simulink model "testNoise"  (R2023b)
settings: Solver=VariableStepAuto  StartTime=0.0  StopTime=10.0  RelTol=1e-3
libraries: simulink x1
settings Model: Creator=grouleau  LastModifiedBy=grouleau

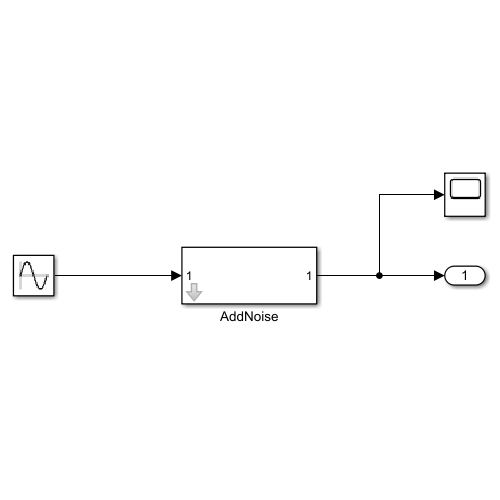
[thumbnail: Simulink's stored preview of the top-level diagram]
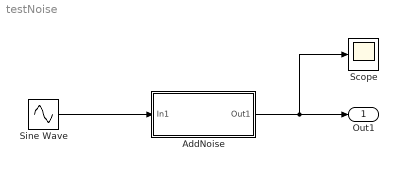
== system testNoise ==
  AddNoise : Subsystem  mask{choice=Random}
      mask prompts: choice "Type of noise"
      mask TypeOptions choice: Random | Pulse | Sequence
  Scope : Scope
  Sine Wave : Sin  Amplitude=5  SampleTime=0
  Out1 : Outport
  wires:
  AddNoise/1(Out1) -> Scope/1, Out1/1
  Sine Wave/1 -> AddNoise/1(In1)

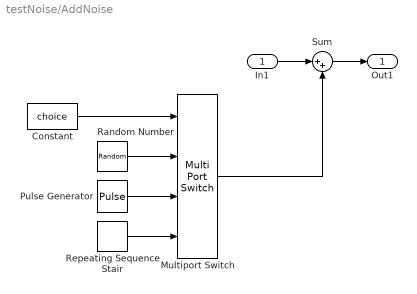
== system testNoise/AddNoise ==
  In1 : Inport
  Constant : Constant  Value=choice
  Multiport Switch : MultiPortSwitch  SaturateOnIntegerOverflow=off  InputSameDT=off
  Pulse Generator : DiscretePulseGenerator  SampleTime=0.1
  Random Number : RandomNumber  SampleTime=0.1
  Repeating Sequence Stair : simulink/Sources/Repeating Sequence Stair  OutValues=[3 1 4 2 1].'  tsamp=0.1  OutMin=[]  OutMax=[]  OutDataTypeStr=double  OutputDataTypeScalingMode=double  OutDataType=fixdt(0,8)  ConRadixGroup=Best Precision: Vector-wise  OutScaling=2^-12
  Sum : Sum  Inputs=|++
  Out1 : Outport
  wires:
  Random Number/1 -> Multiport Switch/2
  Pulse Generator/1 -> Multiport Switch/3
  Repeating Sequence Stair/1 -> Multiport Switch/4
  Sum/1 -> Out1/1
  Multiport Switch/1 -> Sum/2
  In1/1 -> Sum/1
  Constant/1 -> Multiport Switch/1
